simulink model "Project_SADC"  (R2021b)
settings: Solver=ode45  StartTime=0.0  StopTime=T  FixedStep=1e-6  RelTol=1e-12
values from neighbouring files (symbols this model uses):
  A = [A_sc,A_sp]    [Main_SADC_10572571.m]
  Abn0 = Anb0'    [Main_SADC_10572571.m]
  epsilon = deg2rad(23.45)    [Main_SADC_10572571.m]
  m = [0.01 0.05 0.01]'    [Main_SADC_10572571.m]
  N = [n1 n2 n3 n4 n5 n6 n7 n8 n9 n10]    [Main_SADC_10572571.m]
  n_sun = 2*pi / T_sun    (= 1.99238499086e-07)    [Main_SADC_10572571.m]
  P_srp = Fe_tot/c    [Main_SADC_10572571.m]
  R3H0 = data.Re^3*H0    [Main_SADC_10572571.m]
  R_sun = astroConstants(2)    [Main_SADC_10572571.m]
  rho_d = cat(2,ones(1,6)*rho_d_sc,ones(1,4)*rho_d_sp)    [Main_SADC_10572571.m]
  rho_s = cat(2,ones(1,6)*rho_s_sc,ones(1,4)*rho_s_sp)    [Main_SADC_10572571.m]
  ri = [ri_sc,r_sp1,r_sp1,r_sp2,r_sp2]    [Main_SADC_10572571.m]
  w0 = [wx0 wy0 wz0]'    [Main_SADC_10572571.m]
  weights = [0.15;0.5;0.35]    [Main_SADC_10572571.m]
undefined symbols (not defined in the file or in its folder): data, gyro, horizonsensor, magnetometer, rr0, sc, sunsensor, vv0, wheel
libraries: simulink_extras x10
(part 1 of 3)
settings Model: Creator=corra  LastModifiedBy=corra
settings SolverCC: AlgebraicLoopSolver=TrustRegion
settings DebuggingCC: SFMachineParentedDataDiag=warning

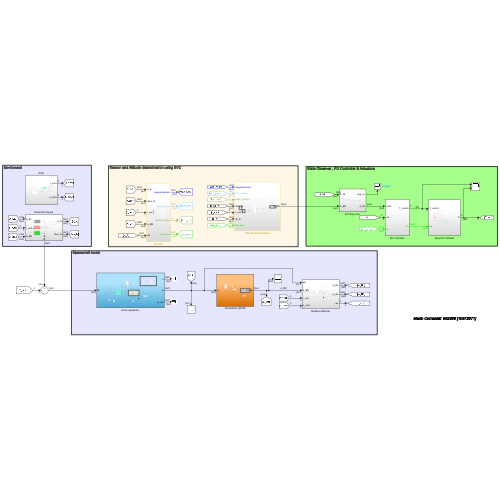
[thumbnail: Simulink's stored preview of the top-level diagram]
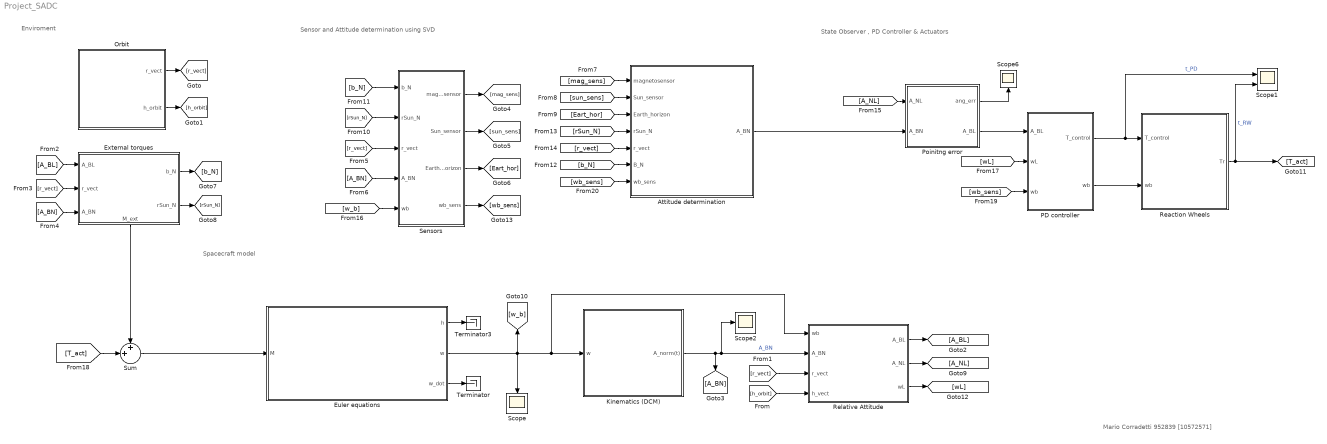
== system Project_SADC ==
  note: Mario Corradetti 952839 [10572571]
  note: Enviroment
  note: State Observer , PD Controller & Actuators
  note: Spacecraft model
  note: Sensor and Attitude determination using SVD
  "Attitude determination " : Subsystem
  Euler equations : Subsystem
  External torques : Subsystem
      settings: PortSchema="{\"entries\":[{\"content\":{\"sides\":[{\"content\":{\"connectorIds\":[\"In1\",\"In2\",\"In3\"]},\"type\":\"ConnectorPlacement.EquallySpacedRectSide\",\"uuid\":\"c5dd5657-11cd-46fc-a813-74747ea81146\"},{\"content\":{\"connectorIds\":[\"Out1\",\"Out2\"],\"side\":\"RIGHT\"},\"type\":\"ConnectorPlacement.EquallySpacedRectSide\",\"uuid\":\"ce8cbc86-0401-4f30-83b3-f262a6771dee\"},{\"content\":{\"connectorIds\":[],\"side\":\"TOP\"},\"type\":\"ConnectorPlacement.EquallySpacedRectSide\",\"uuid\":\"54f7f4d9-1155-478d-825b-4623d6763012\"},{\"content\":{\"connectorIds\":[\"Out3\"],\"side\":\"BOTTOM\"},\"type\":\"ConnectorPlacement.EquallySpacedRectSide\",\"uuid\":\"9bbeb954-f49a-41a5-9c63-5058200ec5df\"}]},\"type\":\"ConnectorPlacement.EquallySpacedConnector\",\"uuid\":\"ae160f86-5b24-4f86-a6f1-a9e1b48113ae\"}],\"packageUris\":[\"http://schema.mathworks.com/mf0/Connector/R2020b\"],\"version\":\"1.0\"}"
  Kinematics (DCM) : Subsystem
  Orbit : Subsystem
  PD controller : Subsystem
  Poinitng error : Subsystem
  Reaction Wheels : Subsystem
  Relative Attitude : Subsystem
  Scope : Scope
  Scope1 : Scope  NumInputPorts=2
  Scope2 : Scope
  Scope6 : Scope
  Sensors : Subsystem
  Sum : Sum  Inputs=++|
  Terminator : Terminator
  Terminator3 : Terminator
  wires:
  Euler equations/3(w_dot) -> Terminator/1
  Orbit/1(r_vect) -> [r_vect]
  Orbit/2(h_orbit) -> [h_orbit]
  Euler equations/1(h) -> Terminator3/1
  Kinematics (DCM)/1(A_norm(t)) -> Scope2/1, Relative Attitude/2(A_BN), [A_BN]  "A_BN"
  [r_vect] -> Relative Attitude/3(r_vect)
  [h_orbit] -> Relative Attitude/4(h_vect)
  Relative Attitude/1(A_BL) -> [A_BL]
  [A_BL] -> External torques/1(A_BL)
  [r_vect] -> External torques/2(r_vect)
  [A_BN] -> External torques/3(A_BN)
  [r_vect] -> Sensors/3(r_vect)
  [A_BN] -> Sensors/4(A_BN)
  Sensors/1(magnetosensor) -> [mag_sens]
  Sensors/2(Sun_sensor) -> [sun_sens]
  Sensors/3(Earth_horizon) -> [Eart_hor]
  [mag_sens] -> "Attitude determination "/1(magnetosensor)
  [sun_sens] -> "Attitude determination "/2(Sun_sensor)
  [Eart_hor] -> "Attitude determination "/3(Earth_horizon)
  External torques/1(b_N) -> [b_N]
  External torques/2(rSun_N) -> [rSun_N]
  [rSun_N] -> Sensors/2(rSun_N)
  [b_N] -> Sensors/1(b_N)
  [b_N] -> "Attitude determination "/6(" B_N ")
  [rSun_N] -> "Attitude determination "/4(rSun_N)
  [r_vect] -> "Attitude determination "/5(r_vect)
  Relative Attitude/2(A_NL) -> [A_NL]
  [A_NL] -> Poinitng error/1(A_NL)
  Poinitng error/1(ang_err) -> Scope6/1
  Poinitng error/2(A_BL) -> PD controller/1(A_BL)
  Euler equations/2(w) -> Scope/1, [w_b], Kinematics (DCM)/1(w), Relative Attitude/1(wb)
  [T_act] -> Sum/2
  Sum/1 -> Euler equations/1(M)
  External torques/3(M_ext) -> Sum/1
  PD controller/1(T_control) -> Reaction Wheels/1(T_control), Scope1/1  "t_PD"
  Relative Attitude/3(wL) -> [wL]
  [wL] -> PD controller/2(" wL ")
  PD controller/2(wb) -> Reaction Wheels/2(wb)
  [w_b] -> Sensors/5(wb)
  Sensors/4(wb_sens) -> [wb_sens]
  Reaction Wheels/1(Tr) -> [T_act], Scope1/2  "t_RW"
  [wb_sens] -> "Attitude determination "/7(wb_sens)
  "Attitude determination "/1(A_BN) -> Poinitng error/2(A_BN)
  [wb_sens] -> PD controller/3("wb ")

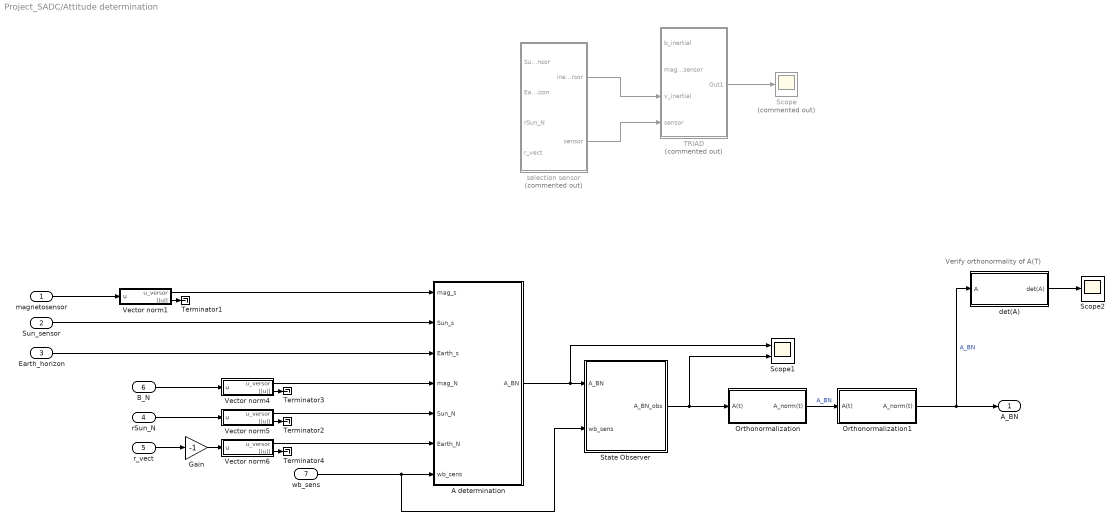
== system Project_SADC/Attitude determination  ==
  note: Verify orthonormality of A(T)
  magnetosensor : Inport
  Sun_sensor : Inport  Port=2
  Earth_horizon : Inport  Port=3
  rSun_N : Inport  Port=4
  r_vect : Inport  Port=5
  " B_N " : Inport  Port=6
  wb_sens : Inport  Port=7
  A determination : Subsystem
  Gain : Gain  Gain=-1
  Orthonormalization : Subsystem
  Orthonormalization1 : Subsystem
  Scope : Scope  Commented=on
  Scope1 : Scope  NumInputPorts=2
  Scope2 : Scope
  State Observer : Subsystem
  "TRIAD " : Subsystem  Commented=on
  Terminator{1..4} (4 alike) : Terminator
  Vector norm1 : Subsystem
  Vector norm4 : Subsystem
  Vector norm5 : Subsystem
  Vector norm6 : Subsystem
  det(A) : Subsystem
  selection sensor : Subsystem  Commented=on
  A_BN : Outport
  wires:
  r_vect/1 -> Gain/1
  magnetosensor/1 -> Vector norm1/1(u)
  Vector norm1/1(u_versor) -> A determination/1(mag_s)
  Sun_sensor/1 -> A determination/2(Sun_s)
  rSun_N/1 -> Vector norm5/1(u)
  Vector norm5/1(u_versor) -> A determination/5(Sun_N)
  Gain/1 -> Vector norm6/1(u)
  Vector norm6/1(u_versor) -> A determination/6(Earth_N)
  Vector norm1/2(||u||) -> Terminator1/1
  Vector norm4/2(||u||) -> Terminator3/1
  Vector norm5/2(||u||) -> Terminator2/1
  Vector norm6/2(||u||) -> Terminator4/1
  Orthonormalization/1(A_norm(t)) -> Orthonormalization1/1(A(t))  "A_BN"
  det(A)/1(det(A)) -> Scope2/1
  selection sensor/1(inertial versor) -> "TRIAD "/3(v_inertial)
  selection sensor/2(sensor) -> "TRIAD "/4(sensor)
  "TRIAD "/1(Out1) -> Scope/1
  " B_N "/1 -> Vector norm4/1(u)
  Vector norm4/1(u_versor) -> A determination/4(mag_N)
  Earth_horizon/1 -> A determination/3(Earth_s)
  wb_sens/1 -> State Observer/2(wb_sens), A determination/7(wb_sens)
  Orthonormalization1/1(A_norm(t)) -> A_BN/1, det(A)/1(A)  "A_BN"
  State Observer/1(A_BN_obs) -> Scope1/2, Orthonormalization/1(A(t))
  A determination/1(A_BN) -> Scope1/1, State Observer/1(A_BN)

== system Project_SADC/Euler equations ==
  note: INERTIA WHEEL
  note: Computation h vector of S/C
  M : Inport
  Clock1 : Clock
  Constant : Constant  Value=sc.I
  Constant1 : Constant  Value=sc.Iinv
  Constant2 : Constant  Value=wheel.I
  Constant3 : Constant  Value=wheel.w
  Gain : Gain  Gain=0
  Integrator : Integrator  InitialCondition=w0
  MatrixMultiply : Product  Multiplication=Matrix(*)
  Product : Product  Multiplication=Matrix(*)
  Product1 : Product  Multiplication=Matrix(*)
  Scope : Scope
  Scope1 : Scope
  Sum : Sum  Inputs=+-
  Sum1 : Sum
  Switch : Switch  Criteria=u2 > Threshold  Threshold=400
  To Workspace : ToWorkspace  VariableName=w  SaveFormat=Timeseries  SampleTime=-1
  product vector : Subsystem
  h : Outport
  w : Outport  Port=2
  w_dot : Outport  Port=3
  wires:
  Sum/1 -> Product1/2
  Product1/1 -> w_dot/1, Integrator/1  "w_dot"
  Product/1 -> h/1, Sum1/2  "h_B"
  Integrator/1 -> To Workspace/1, w/1, product vector/1(A), Product/2  "w"
  Constant1/1 -> Product1/1
  M/1 -> Sum/1  "external_moment & control_moment"
  Constant/1 -> Product/1
  product vector/1(C) -> Sum/2
  Constant2/1 -> MatrixMultiply/1
  Constant3/1 -> MatrixMultiply/2
  Sum1/1 -> Scope1/1, product vector/2(B)
  MatrixMultiply/1 -> Gain/1, Switch/1
  Gain/1 -> Switch/3
  Clock1/1 -> Switch/2
  Switch/1 -> Scope/1, Sum1/1

== system Project_SADC/External torques ==
  A_BL : Inport
  r_vect : Inport  Port=2
  A_BN : Inport  Port=3
  GG torque : Subsystem
  Gain : Gain
  Gain1 : Gain
  Gain2 : Gain
  Magnetic torque : Subsystem
  SRP torque : Subsystem
  Scope : Scope
  Scope1 : Scope
  Sum : Sum  Inputs=+++
  Terminator1 : Terminator
  Vector norm : Subsystem
  b_N : Outport
  rSun_N : Outport  Port=2
  M_ext : Outport  Port=3
  wires:
  A_BL/1 -> GG torque/1(A_BL)
  r_vect/1 -> Magnetic torque/2(r_vect), SRP torque/2(r_vect), GG torque/2(r_vect)
  A_BN/1 -> Magnetic torque/1(A_bn), SRP torque/1(A_BN)
  Sum/1 -> M_ext/1, Vector norm/1(u), Scope/1
  Magnetic torque/1(M_magnetic) -> Gain/1
  SRP torque/1(M_srp) -> Gain1/1
  GG torque/1(M_GG) -> Gain2/1
  Gain/1 -> Sum/1
  Gain1/1 -> Sum/2
  Gain2/1 -> Sum/3
  Magnetic torque/2(b_N) -> b_N/1
  SRP torque/2(rSun_N) -> rSun_N/1
  Vector norm/2(||u||) -> Scope1/1
  Vector norm/1(u_versor) -> Terminator1/1

== system Project_SADC/Kinematics (DCM) ==
  note: Verify orthonormality of A(T)
  w : Inport
  Gain : Gain  Gain=-1
  Integrator : Integrator  InitialCondition=Abn0
  Matrix Multiply : Product  Multiplication=Matrix(*)
  Orthonormalization : Subsystem
  Scope : Scope
  To Workspace : ToWorkspace  VariableName=A_bn  SaveFormat=Timeseries  SampleTime=-1
  det(A) : Subsystem
  w_mat : Subsystem
  A_norm(t) : Outport
  wires:
  w/1 -> w_mat/1(w)
  Matrix Multiply/1 -> Integrator/1  "A_dot"
  Gain/1 -> Matrix Multiply/1
  w_mat/1(w_mat) -> Gain/1
  Integrator/1 -> Orthonormalization/1(A(t))  "A(t)"
  Orthonormalization/1(A_norm(t)) -> det(A)/1(A), To Workspace/1, A_norm(t)/1, Matrix Multiply/2  "A_BN"
  det(A)/1(det(A)) -> Scope/1

== system Project_SADC/Orbit ==
  Constant : Constant  Value=[0 0 0]
  "Orbit integration " : Subsystem
  To Workspace : ToWorkspace  VariableName=h_orbit  SaveFormat=Timeseries  SampleTime=-1
  To Workspace2 : ToWorkspace  VariableName=r_orbit  SaveFormat=Timeseries  SampleTime=-1
  product vector : Subsystem
  r_vect : Outport
  h_orbit : Outport  Port=2
  wires:
  "Orbit integration "/1(r_vect) -> product vector/1(A), r_vect/1, To Workspace2/1
  "Orbit integration "/2(v_vect) -> product vector/2(B)
  Constant/1 -> "Orbit integration "/1(acc_pert)
  product vector/1(C) -> To Workspace/1, h_orbit/1

== system Project_SADC/PD controller ==
  A_BL : Inport
  " wL " : Inport  Port=2
  "wb " : Inport  Port=3
  Clock : Clock
  De-tumbling : Subsystem  TreatAsAtomicUnit=on
  If : If  IfExpression=u1<400
  If Action Subsystem : Subsystem  TreatAsAtomicUnit=on
  Merge : Merge
  T_control : Outport
  wb : Outport  Port=2
  wires:
  A_BL/1 -> If Action Subsystem/1(A_BL)
  If Action Subsystem/1(Output) -> Merge/1
  Merge/1 -> T_control/1
  "wb "/1 -> wb/1, De-tumbling/1(w_b), If Action Subsystem/3(w_b)
  If/1 -> De-tumbling/Action
  If/2 -> If Action Subsystem/Action
  De-tumbling/1(T_ideal) -> Merge/2
  Clock/1 -> If/1
  " wL "/1 -> If Action Subsystem/2("wL  ")

== system Project_SADC/Poinitng error ==
  A_NL : Inport
  A_BN : Inport  Port=2
  Acos : Trigonometry  Operator=acos
  Dot Product : DotProduct  InputSameDT=on  OutDataTypeStr=Inherit: Inherit via internal rule
  MatrixMultiply : Product  Multiplication=Matrix(*)
  MatrixMultiply1 : Product  Multiplication=Matrix(*)
  Radians to Degrees : simulink_extras/Transformations/Radians to Degrees
  To Workspace : ToWorkspace  VariableName=ang_err  SaveFormat=Timeseries  SampleTime=-1
  x_B : Constant  Value=[ 1 0 0 ]
  x_L : Constant  Value=[ 1 0 0 ]
  ang_err : Outport
  A_BL : Outport  Port=2
  wires:
  A_NL/1 -> MatrixMultiply/2
  A_BN/1 -> MatrixMultiply/1
  MatrixMultiply/1 -> A_BL/1, MatrixMultiply1/1  "A_BL"
  x_L/1 -> MatrixMultiply1/2
  MatrixMultiply1/1 -> Dot Product/1  "x_L in B"
  x_B/1 -> Dot Product/2
  Dot Product/1 -> Acos/1
  Acos/1 -> Radians to Degrees/1
  Radians to Degrees/1 -> To Workspace/1, ang_err/1

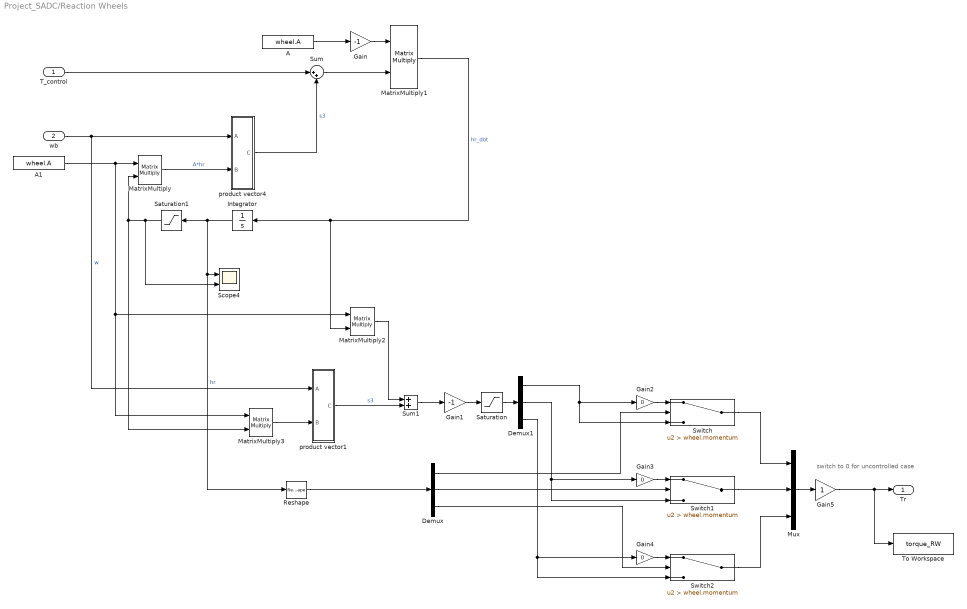
== system Project_SADC/Reaction Wheels ==
  note: switch to 0 for uncontrolled case
  T_control : Inport
  wb : Inport  Port=2
  A : Constant  Value=wheel.A
  A1 : Constant  Value=wheel.A
  Demux : Demux  Outputs=3
  Demux1 : Demux  Outputs=3
  Gain : Gain  Gain=-1
  Gain1 : Gain  Gain=-1
  Gain2 : Gain  Gain=0
  Gain3 : Gain  Gain=0
  Gain4 : Gain  Gain=0
  Gain5 : Gain
  Integrator : Integrator
  MatrixMultiply{,1..3} (4 alike) : Product  Multiplication=Matrix(*)
  Mux : Mux  Inputs=3
  Reshape : Reshape  OutputDimensionality=Column vector (2-D)
  Saturation : Saturate  UpperLimit=wheel.maxtorque  LowerLimit=-wheel.maxtorque  LinearizeAsGain=off
  Saturation1 : Saturate  UpperLimit=wheel.momentum  LowerLimit=-wheel.momentum
  Scope4 : Scope  NumInputPorts=2
  Sum : Sum  Inputs=|++
  Sum1 : Sum
  Switch : Switch  Criteria=u2 > Threshold  Threshold=wheel.momentum
  Switch1 : Switch  Criteria=u2 > Threshold  Threshold=wheel.momentum
  Switch2 : Switch  Criteria=u2 > Threshold  Threshold=wheel.momentum
  To Workspace : ToWorkspace  VariableName=torque_RW  SaveFormat=Timeseries  SampleTime=-1
  product vector1 : Subsystem
  product vector4 : Subsystem
  Tr : Outport
  wires:
  wb/1 -> product vector4/1(A), product vector1/1(A)  "w"
  MatrixMultiply/1 -> product vector4/2(B)  "A*hr"
  Integrator/1 -> Reshape/1, Scope4/1, Saturation1/1  "hr"
  T_control/1 -> Sum/1
  product vector4/1(C) -> Sum/2  "s3"
  MatrixMultiply1/1 -> Integrator/1, MatrixMultiply2/2  "hr_dot"
  Sum/1 -> MatrixMultiply1/2
  A1/1 -> MatrixMultiply3/1, MatrixMultiply2/1, MatrixMultiply/1
  A/1 -> Gain/1
  Gain/1 -> MatrixMultiply1/1
  MatrixMultiply2/1 -> Sum1/1
  product vector1/1(C) -> Sum1/2  "s3"
  Sum1/1 -> Gain1/1
  Gain1/1 -> Saturation/1
  Saturation1/1 -> Scope4/2, MatrixMultiply/2, MatrixMultiply3/2
  MatrixMultiply3/1 -> product vector1/2(B)
  Gain2/1 -> Switch/1
  Demux/1 -> Switch/2
  Gain3/1 -> Switch1/1
  Gain4/1 -> Switch2/1
  Demux/2 -> Switch1/2
  Demux/3 -> Switch2/2
  Switch/1 -> Mux/1
  Switch1/1 -> Mux/2
  Switch2/1 -> Mux/3
  Mux/1 -> Gain5/1
  Reshape/1 -> Demux/1
  Saturation/1 -> Demux1/1
  Demux1/1 -> Switch/3, Gain2/1
  Demux1/2 -> Switch1/3, Gain3/1
  Demux1/3 -> Switch2/3, Gain4/1
  Gain5/1 -> To Workspace/1, Tr/1

== system Project_SADC/Relative Attitude ==
  wb : Inport
  A_BN : Inport  Port=2
  r_vect : Inport  Port=3
  h_vect : Inport  Port=4
  DCM from L to B and from L to N : Subsystem
  MatrixMultiply : Product  Multiplication=Matrix(*)
  Scope : Scope
  Scope1 : Scope
  Sum : Sum  Inputs=-+
  A_BL : Outport
  A_NL : Outport  Port=2
  wL : Outport  Port=3
  wires:
  h_vect/1 -> DCM from L to B and from L to N/3(h_vect)
  DCM from L to B and from L to N/1(A_BL) -> A_BL/1, MatrixMultiply/1
  DCM from L to B and from L to N/2(A_NL) -> A_NL/1
  A_BN/1 -> DCM from L to B and from L to N/1(A_BN)
  Sum/1 -> Scope1/1  "w_B/L"
  r_vect/1 -> DCM from L to B and from L to N/2(r_vect)
  MatrixMultiply/1 -> Sum/1
  wb/1 -> Sum/2
  DCM from L to B and from L to N/3(wL) -> Scope/1, wL/1, MatrixMultiply/2

== system Project_SADC/Sensors ==
  b_N : Inport
  rSun_N : Inport  Port=2
  r_vect : Inport  Port=3
  A_BN : Inport  Port=4
  wb : Inport  Port=5
  Check if in EH FOV : Subsystem
  Check if in sunsensor FOV : Subsystem
  Cylindrical eclipse model : Subsystem  Commented=on
  Earth horizon : Subsystem
  Gyroscope : Subsystem
  Magnetosensor : Subsystem
  MatrixMultiply1 : Product  Multiplication=Matrix(*)
  Scope4 : Scope  NumInputPorts=2
  Scope5 : Scope  NumInputPorts=2
  Scope6 : Scope  NumInputPorts=2
  Sun sensor : Subsystem
  magnetosensor : Outport
  Sun_sensor : Outport  Port=2
  Earth_horizon : Outport  Port=3
  wb_sens : Outport  Port=4
  wires:
  A_BN/1 -> Check if in EH FOV/1(A_BN), MatrixMultiply1/1, Check if in sunsensor FOV/2(A_BN)
  r_vect/1 -> Check if in sunsensor FOV/3(r_vect), Check if in EH FOV/2(r_vect)
  Magnetosensor/1(b_measured) -> Scope4/2, magnetosensor/1
  rSun_N/1 -> Check if in sunsensor FOV/1(rSun_N)
  b_N/1 -> MatrixMultiply1/2
  MatrixMultiply1/1 -> Scope4/1, Magnetosensor/1(b_B)
  Check if in sunsensor FOV/2(rSun_B) -> Sun sensor/1(rSun_B)  "r_sun_B"
  Sun sensor/1(Output1) -> Scope5/2, Sun_sensor/1
  Earth horizon/1(Output2) -> Earth_horizon/1, Scope6/2  "sens"
  wb/1 -> Gyroscope/1(wb)
  Gyroscope/1(w_sens) -> wb_sens/1
  Check if in sunsensor FOV/1(Sun_B) -> Scope5/1
  Check if in EH FOV/1(rvect _B) -> Scope6/1, Earth horizon/1(rEarth_B)  "r_Earth_B"

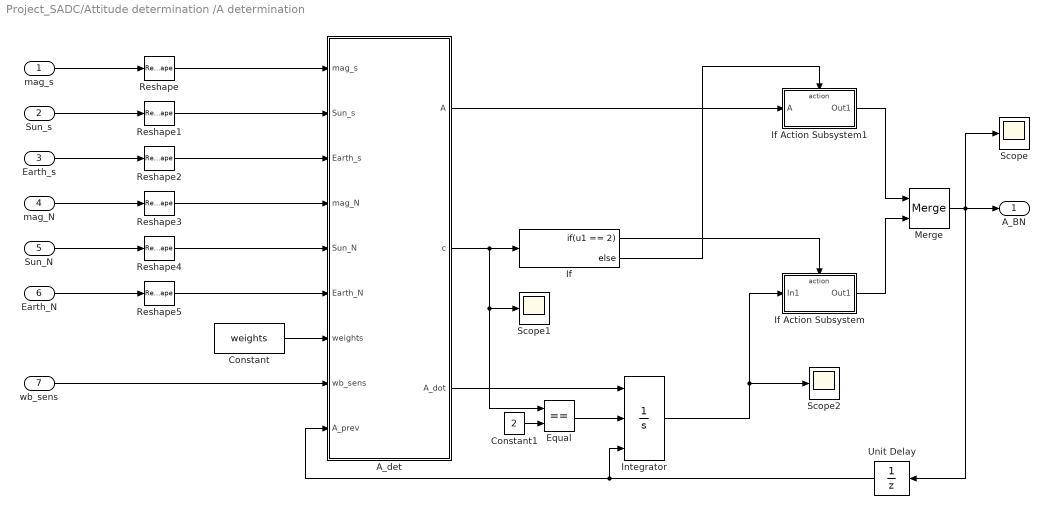
== system Project_SADC/Attitude determination /A determination ==
  mag_s : Inport
  Sun_s : Inport  Port=2
  Earth_s : Inport  Port=3
  mag_N : Inport  Port=4
  Sun_N : Inport  Port=5
  Earth_N : Inport  Port=6
  wb_sens : Inport  Port=7
  A_det : MATLAB Function  TreatAsAtomicUnit=on
  Constant : Constant  Value=weights  VectorParams1D=off
  Constant1 : Constant  Value=2
  Equal : RelationalOperator  Operator===  OutDataTypeStr=boolean  RndMeth=Simplest
  If : If  IfExpression=u1 == 2
  If Action Subsystem : Subsystem  TreatAsAtomicUnit=on
  If Action Subsystem1 : Subsystem  TreatAsAtomicUnit=on
  Integrator : Integrator  ExternalReset=either  InitialConditionSource=external  InitialCondition=eye(3)
  Merge : Merge
  Reshape{,1..5} (6 alike) : Reshape  OutputDimensionality=Column vector (2-D)
  Scope : Scope
  Scope1 : Scope
  Scope2 : Scope
  Unit Delay : UnitDelay  InitialCondition=Abn0  SampleTime=-1  HasFrameUpgradeWarning=on
  A_BN : Outport
  wires:
  mag_s/1 -> Reshape/1
  Sun_s/1 -> Reshape1/1
  Earth_s/1 -> Reshape2/1
  mag_N/1 -> Reshape3/1
  Sun_N/1 -> Reshape4/1
  Earth_N/1 -> Reshape5/1
  Constant/1 -> A_det/7(weights)
  Reshape/1 -> A_det/1(mag_s)
  Reshape1/1 -> A_det/2(Sun_s)
  Reshape2/1 -> A_det/3(Earth_s)
  Reshape3/1 -> A_det/4(mag_N)
  Reshape4/1 -> A_det/5(Sun_N)
  Reshape5/1 -> A_det/6(Earth_N)
  wb_sens/1 -> A_det/8(wb_sens)
  A_det/3(A_dot) -> Integrator/1
  Integrator/1 -> Scope2/1, If Action Subsystem/1(In1)
  A_det/2(c) -> Scope1/1, Equal/1, If/1
  If/1 -> If Action Subsystem/Action
  If/2 -> If Action Subsystem1/Action
  Merge/1 -> Unit Delay/1, Scope/1, A_BN/1
  Equal/1 -> Integrator/2
  Constant1/1 -> Equal/2
  Unit Delay/1 -> A_det/9(A_prev), Integrator/3
  A_det/1(A) -> If Action Subsystem1/1(A)
  If Action Subsystem/1(Out1) -> Merge/2
  If Action Subsystem1/1(Out1) -> Merge/1

== system Project_SADC/Attitude determination /Orthonormalization ==
  A(t) : Inport
  Gain : Gain  Gain=3/2
  Gain1 : Gain  Gain=1/2
  Matrix Multiply : Product  Multiplication=Matrix(*)
  Matrix Multiply1 : Product  Multiplication=Matrix(*)
  Sum : Sum  Inputs=+-
  Transpose : Math  Operator=transpose  SaturateOnIntegerOverflow=on
  A_norm(t) : Outport
  wires:
  Gain/1 -> Sum/1
  Transpose/1 -> Matrix Multiply/2
  A(t)/1 -> Gain/1, Gain1/1, Transpose/1, Matrix Multiply/1
  Matrix Multiply1/1 -> Sum/2
  Sum/1 -> A_norm(t)/1
  Matrix Multiply/1 -> Matrix Multiply1/1
  Gain1/1 -> Matrix Multiply1/2

== system Project_SADC/Attitude determination /Orthonormalization1 ==
  A(t) : Inport
  Gain : Gain  Gain=3/2
  Gain1 : Gain  Gain=1/2
  Matrix Multiply : Product  Multiplication=Matrix(*)
  Matrix Multiply1 : Product  Multiplication=Matrix(*)
  Sum : Sum  Inputs=+-
  Transpose : Math  Operator=transpose  SaturateOnIntegerOverflow=on
  A_norm(t) : Outport
  wires:
  Gain1/1 -> Matrix Multiply1/2
  Matrix Multiply/1 -> Matrix Multiply1/1
  Sum/1 -> A_norm(t)/1
  Matrix Multiply1/1 -> Sum/2
  A(t)/1 -> Matrix Multiply/1, Transpose/1, Gain1/1, Gain/1
  Transpose/1 -> Matrix Multiply/2
  Gain/1 -> Sum/1

== system Project_SADC/Attitude determination /State Observer ==
  A_BN : Inport
  wb_sens : Inport  Port=2
  Gain : Gain  Gain=-0.6
  Gain1 : Gain  Gain=+1
  Integrator1 : Integrator  InitialCondition=Abn0
  MatrixMultiply : Product  Multiplication=Matrix(*)
  Scope : Scope  NumInputPorts=2
  Subsystem : Subsystem
  Sum : Sum  Inputs=|++
  Sum1 : Sum  Inputs=+-
  A_BN_obs : Outport
  wires:
  Integrator1/1 -> Scope/1, A_BN_obs/1, MatrixMultiply/2, Sum1/1  "ABN_obs"
  Subsystem/1(skew_mat) -> Gain1/1
  A_BN/1 -> Scope/2, Sum1/2  "ABN_sens"
  Sum1/1 -> Gain/1
  MatrixMultiply/1 -> Sum/1
  Gain/1 -> Sum/2
  Sum/1 -> Integrator1/1
  wb_sens/1 -> Subsystem/1(vect)  "wb_obs"
  Gain1/1 -> MatrixMultiply/1

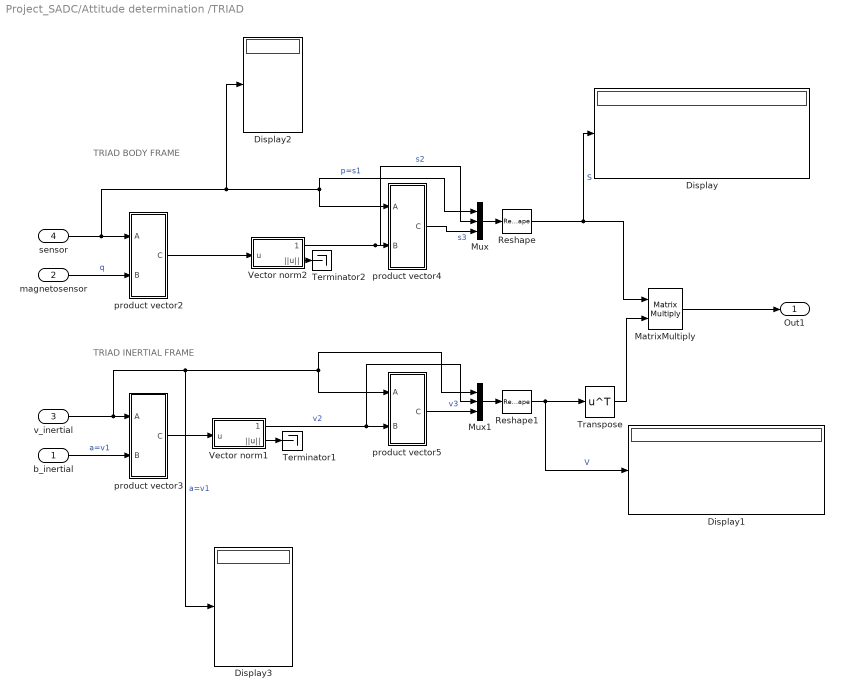
== system Project_SADC/Attitude determination /TRIAD  ==
  note: TRIAD BODY FRAME
  note: TRIAD INERTIAL FRAME
  b_inertial : Inport
  magnetosensor : Inport  Port=2
  v_inertial : Inport  Port=3
  sensor : Inport  Port=4
  Display{,1..3} (4 alike) : Display
  MatrixMultiply : Product  Multiplication=Matrix(*)
  Mux : Mux  Inputs=3
  Mux1 : Mux  Inputs=3
  Reshape : Reshape  OutputDimensionality=Customize  OutputDimensions=[3,3]
  Reshape1 : Reshape  OutputDimensionality=Customize  OutputDimensions=[3,3]
  Terminator1 : Terminator
  Terminator2 : Terminator
  Transpose : Math  Operator=transpose  SaturateOnIntegerOverflow=on
  Vector norm1 : Subsystem
  Vector norm2 : Subsystem
  product vector2 : Subsystem
  product vector3 : Subsystem
  product vector4 : Subsystem
  product vector5 : Subsystem
  Out1 : Outport
  wires:
  sensor/1 -> Display2/1, Mux/1, product vector4/1(A), product vector2/1(A)  "p=s1"
  magnetosensor/1 -> product vector2/2(B)  "q"
  v_inertial/1 -> Display3/1, Mux1/1, product vector5/1(A), product vector3/1(A)  "a=v1"
  product vector2/1(C) -> Vector norm2/1(u)
  product vector3/1(C) -> Vector norm1/1(u)
  Vector norm2/1(u_versor) -> Mux/2, product vector4/2(B)  "s2"
  Vector norm1/1(u_versor) -> Mux1/2, product vector5/2(B)  "v2"
  product vector5/1(C) -> Mux1/3  "v3"
  product vector4/1(C) -> Mux/3  "s3"
  Mux/1 -> Reshape/1
  Mux1/1 -> Reshape1/1
  Reshape/1 -> Display/1, MatrixMultiply/1  "S"
  Reshape1/1 -> Display1/1, Transpose/1  "V"
  MatrixMultiply/1 -> Out1/1
  Transpose/1 -> MatrixMultiply/2
  Vector norm2/2(||u||) -> Terminator2/1
  Vector norm1/2(||u||) -> Terminator1/1
  b_inertial/1 -> product vector3/2(B)  "a=v1"

== system Project_SADC/Attitude determination /Vector norm1 ==
  u : Inport
  Divide : Product  Inputs=*/
  norm_vector : Subsystem
  u_versor : Outport
  ||u|| : Outport  Port=2
  wires:
  u/1 -> Divide/1, norm_vector/1(u)
  norm_vector/1(|u|) -> ||u||/1, Divide/2
  Divide/1 -> u_versor/1

== system Project_SADC/Attitude determination /Vector norm4 ==
  u : Inport
  Divide : Product  Inputs=*/
  norm_vector : Subsystem
  u_versor : Outport
  ||u|| : Outport  Port=2
  wires:
  u/1 -> Divide/1, norm_vector/1(u)
  norm_vector/1(|u|) -> ||u||/1, Divide/2
  Divide/1 -> u_versor/1

== system Project_SADC/Attitude determination /Vector norm5 ==
  u : Inport
  Divide : Product  Inputs=*/
  norm_vector : Subsystem
  u_versor : Outport
  ||u|| : Outport  Port=2
  wires:
  Divide/1 -> u_versor/1
  norm_vector/1(|u|) -> Divide/2, ||u||/1
  u/1 -> norm_vector/1(u), Divide/1

== system Project_SADC/Attitude determination /Vector norm6 ==
  u : Inport
  Divide : Product  Inputs=*/
  norm_vector : Subsystem
  u_versor : Outport
  ||u|| : Outport  Port=2
  wires:
  u/1 -> Divide/1, norm_vector/1(u)
  norm_vector/1(|u|) -> ||u||/1, Divide/2
  Divide/1 -> u_versor/1

== system Project_SADC/Attitude determination /det(A) ==
  A : Inport
  Demux : Demux  Outputs=9
  Product{,1..8} (9 alike) : Product
  Reshape : Reshape  OutputDimensionality=Customize  OutputDimensions=[9,1]
  Sum : Sum  Inputs=+-
  Sum1 : Sum  Inputs=+-+
  Sum2 : Sum  Inputs=+-
  Sum3 : Sum  Inputs=+-
  det(A) : Outport
  wires:
  Product/1 -> Sum/1
  Demux/5 -> Product7/1, Product/1  "a22"
  Demux/9 -> Product3/2, Product/2  "a33"
  Demux/6 -> Product1/1, Product4/2  "a23"
  Demux/8 -> Product1/2, Product6/2  "a32"
  Product1/1 -> Sum/2
  Demux/1 -> Product2/2  "a11"
  Sum/1 -> Product2/1
  Demux/4 -> Product6/1, Product3/1  "a21"
  Demux/7 -> Product7/2, Product4/1  "a31"
  Product3/1 -> Sum2/1
  Product4/1 -> Sum2/2
  Sum2/1 -> Product5/2
  Demux/2 -> Product5/1  "a12"
  Product2/1 -> Sum1/1
  Product5/1 -> Sum1/2
  Product6/1 -> Sum3/1
  Product7/1 -> Sum3/2
  Sum3/1 -> Product8/2
  Demux/3 -> Product8/1  "a13"
  Product8/1 -> Sum1/3
  Sum1/1 -> det(A)/1
  Reshape/1 -> Demux/1
  A/1 -> Reshape/1

== system Project_SADC/Attitude determination /selection sensor ==
  Sun_sensor : Inport
  Earth_horizon : Inport  Port=2
  rSun_N : Inport  Port=3
  r_vect : Inport  Port=4
  If : If  IfExpression=u1==0
  If Action Subsystem : Subsystem  TreatAsAtomicUnit=on
  If Action Subsystem1 : Subsystem  TreatAsAtomicUnit=on
  If Action Subsystem2 : Subsystem  TreatAsAtomicUnit=on
  If Action Subsystem3 : Subsystem  TreatAsAtomicUnit=on
  If1 : If  IfExpression=u1==0
  Merge : Merge
  Merge1 : Merge
  Terminator : Terminator
  Vector norm3 : Subsystem
  inertial versor : Outport
  sensor : Outport  Port=2
  wires:
  Sun_sensor/1 -> If Action Subsystem1/1(Sun_sensor), Vector norm3/1(u)
  If/1 -> If Action Subsystem/Action
  If/2 -> If Action Subsystem1/Action
  Earth_horizon/1 -> If Action Subsystem/1(Earth_horizon)
  Vector norm3/2(||u||) -> If1/1, If/1
  Vector norm3/1(u_versor) -> Terminator/1
  If Action Subsystem1/1(Out1) -> Merge/2
  If Action Subsystem/1(Out1) -> Merge/1
  Merge/1 -> sensor/1
  r_vect/1 -> If Action Subsystem2/1(r_vect)
  rSun_N/1 -> If Action Subsystem3/1(In1)
  If Action Subsystem2/1(Out1) -> Merge1/1
  If Action Subsystem3/1(Out1) -> Merge1/2
  Merge1/1 -> inertial versor/1
  If1/1 -> If Action Subsystem2/Action
  If1/2 -> If Action Subsystem3/Action

== system Project_SADC/Euler equations/product vector ==
  A : Inport
  B : Inport  Port=2
  Mux : Mux  Inputs=3
  i-component : Subsystem
  j-component : Subsystem
  k-component1 : Subsystem
  C : Outport
  wires:
  Mux/1 -> C/1
  A/1 -> k-component1/1(A), j-component/1(A), i-component/1(A)
  B/1 -> k-component1/2(B), j-component/2(B), i-component/2(B)
  i-component/1(Out2) -> Mux/1
  j-component/1(Out1) -> Mux/2
  k-component1/1(Out1) -> Mux/3

== system Project_SADC/External torques/GG torque ==
  A_BL : Inport
  r_vect : Inport  Port=2
  Constant : Constant  Value=-3
  Constant1 : Constant  Value=[1 0 0]'  VectorParams1D=off
  Constant2 : Constant  Value=sc.I  VectorParams1D=off
  Gain : Gain  Gain=data.mu*3
  MatrixMultiply : Product  Multiplication=Matrix(*)
  MatrixMultiply1 : Product  Multiplication=Matrix(*)
  MatrixMultiply2 : Product  Multiplication=Matrix(*)
  Power : Math  Operator=pow  SaturateOnIntegerOverflow=on
  Reshape : Reshape  OutputDimensionality=Column vector (2-D)
  Scope : Scope
  Terminator : Terminator
  To Workspace : ToWorkspace  VariableName=M_GG  SaveFormat=Timeseries  SampleTime=-1
  Vector norm : Subsystem
  product vector : Subsystem
  M_GG : Outport
  wires:
  r_vect/1 -> Vector norm/1(u)
  Vector norm/1(u_versor) -> Terminator/1
  Vector norm/2(||u||) -> Power/1
  Constant/1 -> Power/2
  Power/1 -> Gain/1
  A_BL/1 -> MatrixMultiply/1
  Constant1/1 -> MatrixMultiply/2
  MatrixMultiply/1 -> product vector/1(A), MatrixMultiply1/2  "[c1,c2,c3]'"
  Constant2/1 -> MatrixMultiply1/1
  MatrixMultiply1/1 -> product vector/2(B)
  Gain/1 -> MatrixMultiply2/2
  product vector/1(C) -> MatrixMultiply2/1
  MatrixMultiply2/1 -> Reshape/1
  Reshape/1 -> To Workspace/1, Scope/1, M_GG/1

== system Project_SADC/External torques/Magnetic torque ==
  A_bn : Inport
  r_vect : Inport  Port=2
  Clock : Clock
  Constant : Constant  Value=m
  MatrixMultiply : Product  Multiplication=Matrix(*)
  Reshape : Reshape  OutputDimensionality=Column vector (2-D)
  Scope : Scope
  To Workspace : ToWorkspace  VariableName=M_magnetic  SaveFormat=Timeseries  SampleTime=-1
  mag_field in inertial : Subsystem
  product vector2 : Subsystem
  M_magnetic : Outport
  b_N : Outport  Port=2
  wires:
  r_vect/1 -> mag_field in inertial/1(r_vect)
  Clock/1 -> mag_field in inertial/2(time)
  mag_field in inertial/1(b_B) -> b_N/1, MatrixMultiply/2
  A_bn/1 -> MatrixMultiply/1
  MatrixMultiply/1 -> product vector2/2(B)  "magnetic vector in body frame"
  Constant/1 -> product vector2/1(A)
  product vector2/1(C) -> Reshape/1
  Reshape/1 -> To Workspace/1, Scope/1, M_magnetic/1

== system Project_SADC/External torques/SRP torque ==
  A_BN : Inport
  r_vect : Inport  Port=2
  Clock : Clock
  Display : Display
  SRP forces : Subsystem
  Scope : Scope
  Scope1 : Scope
  Sun wrt s/c : Subsystem
  To Workspace : ToWorkspace  VariableName=M_srp  SaveFormat=Timeseries  SampleTime=-1
  Torques on faces of s/c : Subsystem
  M_srp : Outport
  rSun_N : Outport  Port=2
  wires:
  A_BN/1 -> Sun wrt s/c/1(A_BN)
  r_vect/1 -> Sun wrt s/c/2(r_vect)
  Clock/1 -> Sun wrt s/c/3(t)
  Sun wrt s/c/1(r_sun) -> Display/1, SRP forces/1(r_Sun)  "r_Sun_in_body"
  SRP forces/2(S_dot_N) -> Torques on faces of s/c/2(S_N)
  SRP forces/1(F_srp) -> Torques on faces of s/c/1(F_srp), Scope/1
  Sun wrt s/c/2(rSun_N) -> rSun_N/1
  Torques on faces of s/c/1(M_srp) -> Scope1/1, To Workspace/1, M_srp/1  "M_srp"

== system Project_SADC/External torques/Vector norm ==
  u : Inport
  Divide : Product  Inputs=*/
  norm_vector : Subsystem
  u_versor : Outport
  ||u|| : Outport  Port=2
  wires:
  u/1 -> Divide/1, norm_vector/1(u)
  norm_vector/1(|u|) -> ||u||/1, Divide/2
  Divide/1 -> u_versor/1

== system Project_SADC/Kinematics (DCM)/Orthonormalization ==
  A(t) : Inport
  Gain : Gain  Gain=3/2
  Gain1 : Gain  Gain=1/2
  Matrix Multiply : Product  Multiplication=Matrix(*)
  Matrix Multiply1 : Product  Multiplication=Matrix(*)
  Sum : Sum  Inputs=+-
  Transpose : Math  Operator=transpose  SaturateOnIntegerOverflow=on
  A_norm(t) : Outport
  wires:
  Gain/1 -> Sum/1
  Transpose/1 -> Matrix Multiply/2
  A(t)/1 -> Gain/1, Gain1/1, Transpose/1, Matrix Multiply/1
  Matrix Multiply1/1 -> Sum/2
  Sum/1 -> A_norm(t)/1
  Matrix Multiply/1 -> Matrix Multiply1/1
  Gain1/1 -> Matrix Multiply1/2

== system Project_SADC/Kinematics (DCM)/det(A) ==
  A : Inport
  Demux : Demux  Outputs=9
  Product{,1..8} (9 alike) : Product
  Reshape : Reshape  OutputDimensionality=Customize  OutputDimensions=[9,1]
  Sum : Sum  Inputs=+-
  Sum1 : Sum  Inputs=+-+
  Sum2 : Sum  Inputs=+-
  Sum3 : Sum  Inputs=+-
  det(A) : Outport
  wires:
  Product/1 -> Sum/1
  Demux/5 -> Product7/1, Product/1  "a22"
  Demux/9 -> Product3/2, Product/2  "a33"
  Demux/6 -> Product1/1, Product4/2  "a23"
  Demux/8 -> Product1/2, Product6/2  "a32"
  Product1/1 -> Sum/2
  Demux/1 -> Product2/2  "a11"
  Sum/1 -> Product2/1
  Demux/4 -> Product6/1, Product3/1  "a21"
  Demux/7 -> Product7/2, Product4/1  "a31"
  Product3/1 -> Sum2/1
  Product4/1 -> Sum2/2
  Sum2/1 -> Product5/2
  Demux/2 -> Product5/1  "a12"
  Product2/1 -> Sum1/1
  Product5/1 -> Sum1/2
  Product6/1 -> Sum3/1
  Product7/1 -> Sum3/2
  Sum3/1 -> Product8/2
  Demux/3 -> Product8/1  "a13"
  Product8/1 -> Sum1/3
  Sum1/1 -> det(A)/1
  Reshape/1 -> Demux/1
  A/1 -> Reshape/1

== system Project_SADC/Kinematics (DCM)/w_mat ==
  w : Inport
  Constant : Constant  Value=0
  Constant1 : Constant  Value=0
  Constant7 : Constant  Value=0
  Demux : Demux  Outputs=3
  Gain1 : Gain  Gain=-1
  Gain2 : Gain  Gain=-1
  Gain3 : Gain  Gain=-1
  Mux : Mux  Inputs=9
  Reshape : Reshape  OutputDimensionality=Customize  OutputDimensions=[3,3]
  Transpose : Math  Operator=transpose  SaturateOnIntegerOverflow=on
  w_mat : Outport
  wires:
  Gain3/1 -> Mux/7
  Demux/2 -> Mux/3, Gain3/1
  Demux/3 -> Mux/4, Gain2/1
  Constant7/1 -> Mux/9
  Demux/1 -> Mux/8, Gain1/1
  Constant/1 -> Mux/1
  Mux/1 -> Reshape/1
  Constant1/1 -> Mux/5
  Gain2/1 -> Mux/2
  Gain1/1 -> Mux/6
  w/1 -> Demux/1
  Reshape/1 -> Transpose/1
  Transpose/1 -> w_mat/1

== system Project_SADC/Orbit/Orbit integration  ==
  acc_pert : Inport
  Constant : Constant  Value=-3
  Gain : Gain  Gain=- data.mu
  Integrator : Integrator  InitialCondition=vv0
  Integrator1 : Integrator  InitialCondition=rr0
  MatrixMultiply : Product
  Power : Math  Operator=pow  SaturateOnIntegerOverflow=on
  Subsystem1 : Subsystem
  Sum : Sum  Inputs=|++
  Terminator : Terminator
  r_vect : Outport
  v_vect : Outport  Port=2
  wires:
  Integrator/1 -> v_vect/1, Integrator1/1  "v"
  Integrator1/1 -> MatrixMultiply/1, Subsystem1/1(u), r_vect/1  "r"
  acc_pert/1 -> Sum/1
  Sum/1 -> Integrator/1  "a"
  Gain/1 -> Sum/2
  Subsystem1/2(||u||) -> Power/1  "||r||"
  Subsystem1/1(u_versor) -> Terminator/1
  Constant/1 -> Power/2
  MatrixMultiply/1 -> Gain/1
  Power/1 -> MatrixMultiply/2  "||r||^-3"

== system Project_SADC/Orbit/product vector ==
  A : Inport
  B : Inport  Port=2
  Mux : Mux  Inputs=3
  i-component : Subsystem
  j-component : Subsystem
  k-component1 : Subsystem
  C : Outport
  wires:
  Mux/1 -> C/1
  A/1 -> k-component1/1(A), j-component/1(A), i-component/1(A)
  B/1 -> k-component1/2(B), j-component/2(B), i-component/2(B)
  i-component/1(Out2) -> Mux/1
  j-component/1(Out1) -> Mux/2
  k-component1/1(Out1) -> Mux/3

== system Project_SADC/PD controller/De-tumbling ==
  note: Proportional
  w_b : Inport
  Action Port : ActionPort  ActionPortLabel=if(u1<400)
  Demux : Demux  Outputs=3
  Mux2 : Mux  Inputs=3
  kd1 : Gain  Gain=-1e-3
  kd2 : Gain  Gain=-1e-3
  kp : Gain  Gain=-1e-3
  T_ideal : Outport
  wires:
  Demux/1 -> kd2/1
  kd2/1 -> Mux2/1
  kp/1 -> Mux2/3
  Demux/2 -> kd1/1
  Demux/3 -> kp/1
  kd1/1 -> Mux2/2
  w_b/1 -> Demux/1
  Mux2/1 -> T_ideal/1

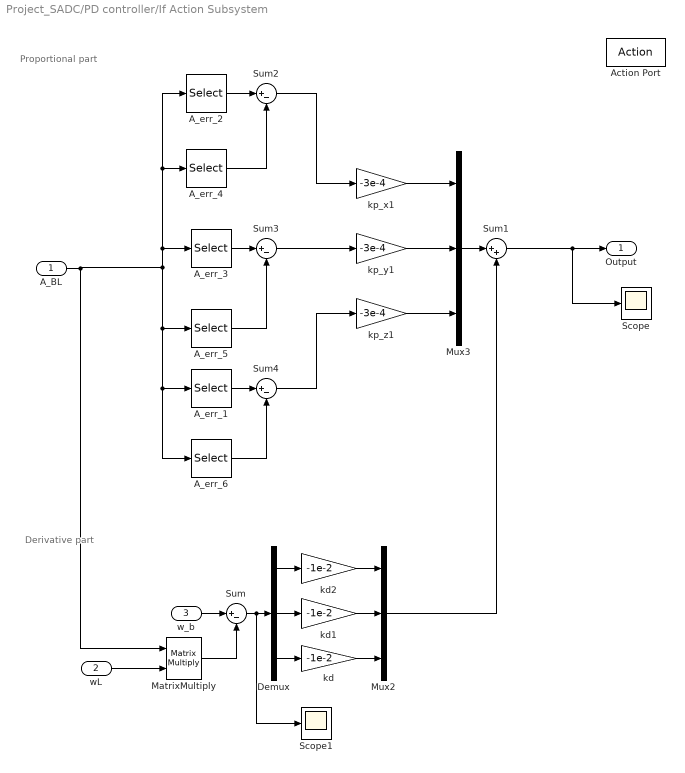
== system Project_SADC/PD controller/If Action Subsystem ==
  note: Derivative part
  note: Proportional part
  A_BL : Inport
  "wL  " : Inport  Port=2
  w_b : Inport  Port=3
  Action Port : ActionPort  ActionPortLabel=else
  A_err_1 : Selector  NumberOfDimensions=2  InputPortWidth=3  IndexOptions=Index vector (dialog),Index vector (dialog)  Indices=1,2  OutputSizes=1,1
  A_err_2 : Selector  NumberOfDimensions=2  InputPortWidth=3  IndexOptions=Index vector (dialog),Index vector (dialog)  Indices=2,3  OutputSizes=1,1
  A_err_3 : Selector  NumberOfDimensions=2  InputPortWidth=3  IndexOptions=Index vector (dialog),Index vector (dialog)  Indices=3,1  OutputSizes=1,1
  A_err_4 : Selector  NumberOfDimensions=2  InputPortWidth=3  IndexOptions=Index vector (dialog),Index vector (dialog)  Indices=3,2  OutputSizes=1,1
  A_err_5 : Selector  NumberOfDimensions=2  InputPortWidth=3  IndexOptions=Index vector (dialog),Index vector (dialog)  Indices=1,3  OutputSizes=1,1
  A_err_6 : Selector  NumberOfDimensions=2  InputPortWidth=3  IndexOptions=Index vector (dialog),Index vector (dialog)  Indices=2,1  OutputSizes=1,1
  Demux : Demux  Outputs=3
  MatrixMultiply : Product  Multiplication=Matrix(*)
  Mux2 : Mux  Inputs=3
  Mux3 : Mux  Inputs=3
  Scope : Scope
  Scope1 : Scope
  Sum{,2..4} (4 alike) : Sum  Inputs=|+-
  Sum1 : Sum  Inputs=|++
  kd : Gain  Gain=-1e-2
  kd1 : Gain  Gain=-1e-2
  kd2 : Gain  Gain=-1e-2
  kp_x1 : Gain  Gain=-3e-4
  kp_y1 : Gain  Gain=-3e-4
  kp_z1 : Gain  Gain=-3e-4
  Output : Outport
  wires:
  MatrixMultiply/1 -> Sum/2
  kd/1 -> Mux2/3
  kd1/1 -> Mux2/2
  Demux/1 -> kd2/1
  Mux2/1 -> Sum1/2
  Demux/3 -> kd/1
  w_b/1 -> Sum/1
  Sum/1 -> Scope1/1, Demux/1
  kd2/1 -> Mux2/1
  Demux/2 -> kd1/1
  "wL  "/1 -> MatrixMultiply/2
  Sum1/1 -> Output/1, Scope/1
  kp_x1/1 -> Mux3/1
  kp_y1/1 -> Mux3/2
  kp_z1/1 -> Mux3/3
  A_BL/1 -> A_err_4/1, A_err_2/1, A_err_3/1, A_err_5/1, A_err_6/1, A_err_1/1, MatrixMultiply/1
  Mux3/1 -> Sum1/1
  A_err_2/1 -> Sum2/1
  A_err_4/1 -> Sum2/2
  A_err_3/1 -> Sum3/1
  A_err_5/1 -> Sum3/2
  A_err_1/1 -> Sum4/1
  A_err_6/1 -> Sum4/2
  Sum2/1 -> kp_x1/1
  Sum3/1 -> kp_y1/1
  Sum4/1 -> kp_z1/1

== system Project_SADC/Reaction Wheels/product vector1 ==
  A : Inport
  B : Inport  Port=2
  Mux : Mux  Inputs=3
  i-component : Subsystem
  j-component : Subsystem
  k-component1 : Subsystem
  C : Outport
  wires:
  k-component1/1(Out1) -> Mux/3
  j-component/1(Out1) -> Mux/2
  i-component/1(Out2) -> Mux/1
  B/1 -> i-component/2(B), j-component/2(B), k-component1/2(B)
  A/1 -> i-component/1(A), j-component/1(A), k-component1/1(A)
  Mux/1 -> C/1

== system Project_SADC/Reaction Wheels/product vector4 ==
  A : Inport
  B : Inport  Port=2
  Mux : Mux  Inputs=3
  i-component : Subsystem
  j-component : Subsystem
  k-component1 : Subsystem
  C : Outport
  wires:
  Mux/1 -> C/1
  A/1 -> k-component1/1(A), j-component/1(A), i-component/1(A)
  B/1 -> k-component1/2(B), j-component/2(B), i-component/2(B)
  i-component/1(Out2) -> Mux/1
  j-component/1(Out1) -> Mux/2
  k-component1/1(Out1) -> Mux/3

== system Project_SADC/Relative Attitude/DCM from L to B and from L to N ==
  A_BN : Inport
  r_vect : Inport  Port=2
  h_vect : Inport  Port=3
  DCM from L to N : Subsystem
  Divide : Product  Inputs=*/
  Gain : Gain  Gain=[ 0 0 1]
  MatrixMultiply : Product  Multiplication=Matrix(*)
  Square : Math  Operator=square  SaturateOnIntegerOverflow=on
  Terminator1 : Terminator
  Terminator2 : Terminator
  To Workspace : ToWorkspace  VariableName=A_nl  SaveFormat=Timeseries  SampleTime=-1
  Vector norm : Subsystem
  Vector norm1 : Subsystem
  A_BL : Outport
  A_NL : Outport  Port=2
  wL : Outport  Port=3
  wires:
  DCM from L to N/1(A_NL) -> To Workspace/1, A_NL/1, MatrixMultiply/2  "A_NL"
  MatrixMultiply/1 -> A_BL/1  "A_BL"
  A_BN/1 -> MatrixMultiply/1
  h_vect/1 -> Vector norm1/1(u), DCM from L to N/2(h_vect)  "h"
  Vector norm/1(u_versor) -> Terminator2/1
  r_vect/1 -> DCM from L to N/1(r_vect), Vector norm/1(u)  "r"
  Divide/1 -> Gain/1  "wL"
  Square/1 -> Divide/2
  Vector norm/2(||u||) -> Square/1
  Vector norm1/2(||u||) -> Divide/1
  Vector norm1/1(u_versor) -> Terminator1/1
  Gain/1 -> wL/1

== system Project_SADC/Sensors/Check if in EH FOV ==
  A_BN : Inport
  r_vect : Inport  Port=2
  Acos : Trigonometry  Operator=acos
  Constant : Constant  Value=[-1 0 0]
  Dot Product : DotProduct  InputSameDT=on  OutDataTypeStr=Inherit: Inherit via internal rule
  Gain : Gain  Gain=-1
  If : If  IfExpression=u1 > 90
  If Action Subsystem : Subsystem  TreatAsAtomicUnit=on
  If Action Subsystem1 : Subsystem  TreatAsAtomicUnit=on
  MatrixMultiply : Product  Multiplication=Matrix(*)
  Merge : Merge
  Radians to Degrees : simulink_extras/Transformations/Radians to Degrees
  Scope : Scope
  Terminator : Terminator
  Vector norm1 : Subsystem
  rvect _B : Outport
  wires:
  MatrixMultiply/1 -> Vector norm1/1(u)
  Vector norm1/1(u_versor) -> If Action Subsystem1/1(u_versor), If Action Subsystem/1(u_versor), Dot Product/1
  Radians to Degrees/1 -> If/1, Scope/1
  Merge/1 -> rvect _B/1
  If Action Subsystem/1(Out1) -> Merge/1
  If Action Subsystem1/1(Out1) -> Merge/2
  If/2 -> If Action Subsystem1/Action
  If/1 -> If Action Subsystem/Action
  Constant/1 -> Dot Product/2
  Acos/1 -> Radians to Degrees/1
  Dot Product/1 -> Acos/1
  Vector norm1/2(||u||) -> Terminator/1
  A_BN/1 -> MatrixMultiply/1
  Gain/1 -> MatrixMultiply/2  "r_vect_in_N"
  r_vect/1 -> Gain/1

== system Project_SADC/Sensors/Check if in sunsensor FOV ==
  rSun_N : Inport
  A_BN : Inport  Port=2
  r_vect : Inport  Port=3
  Acos : Trigonometry  Operator=acos
  Constant : Constant  Value=[1 0 0]
  Dot Product : DotProduct  InputSameDT=on  OutDataTypeStr=Inherit: Inherit via internal rule
  Gain : Gain  Gain=-1
  If : If  IfExpression=u1 > 60
  If Action Subsystem : Subsystem  TreatAsAtomicUnit=on
  If Action Subsystem1 : Subsystem  TreatAsAtomicUnit=on
  MatrixMultiply : Product  Multiplication=Matrix(*)
  MatrixMultiply1 : Product  Multiplication=Matrix(*)
  Merge : Merge
  Radians to Degrees : simulink_extras/Transformations/Radians to Degrees
  Scope : Scope
  Sum : Sum  Inputs=|++
  Terminator : Terminator
  Vector norm1 : Subsystem
  Sun_B : Outport
  rSun_B : Outport  Port=2
  wires:
  r_vect/1 -> Gain/1
  Sum/1 -> MatrixMultiply/2  "r_sun_sc_in_N"
  A_BN/1 -> MatrixMultiply1/1, MatrixMultiply/1
  Vector norm1/2(||u||) -> Terminator/1
  MatrixMultiply/1 -> Vector norm1/1(u)
  Dot Product/1 -> Acos/1
  Acos/1 -> Radians to Degrees/1
  Constant/1 -> Dot Product/2
  rSun_N/1 -> MatrixMultiply1/2, Sum/1
  Gain/1 -> Sum/2
  If/1 -> If Action Subsystem/Action
  If/2 -> If Action Subsystem1/Action
  If Action Subsystem1/1(Out1) -> Merge/2
  If Action Subsystem/1(Out1) -> Merge/1
  Merge/1 -> rSun_B/1
  Radians to Degrees/1 -> Scope/1, If/1
  Vector norm1/1(u_versor) -> Dot Product/1
  MatrixMultiply1/1 -> Sun_B/1, If Action Subsystem1/1(In1), If Action Subsystem/1(In1)

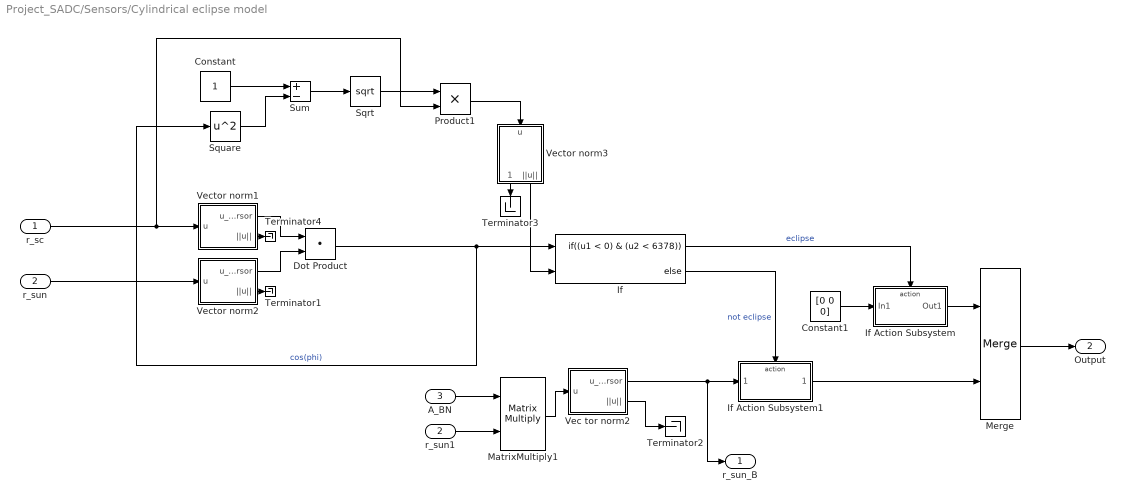
== system Project_SADC/Sensors/Cylindrical eclipse model ==
  r_sc : Inport
  r_sun : Inport  Port=2
  A_BN : Inport  Port=3
  Constant : Constant
  Constant1 : Constant  Value=[0 0 0]
  Dot Product : DotProduct  InputSameDT=on  OutDataTypeStr=Inherit: Inherit via internal rule
  If : If  NumInputs=2  IfExpression=(u1 < 0) & (u2 < 6378)
  If Action Subsystem : Subsystem  TreatAsAtomicUnit=on
  If Action Subsystem1 : Subsystem  TreatAsAtomicUnit=on
  MatrixMultiply1 : Product  Multiplication=Matrix(*)
  Merge : Merge
  Product1 : Product
  Sqrt : Sqrt  SaturateOnIntegerOverflow=on
  Square : Math  Operator=square  SaturateOnIntegerOverflow=on
  Sum : Sum  Inputs=+-
  Terminator{1..4} (4 alike) : Terminator
  Vec tor norm2 : Subsystem
  Vector norm1 : Subsystem
  Vector norm2 : Subsystem
  Vector norm3 : Subsystem
  r_sun1 : InportShadow  Port=2
  r_sun_B : Outport
  Output : Outport  Port=2
  wires:
  r_sc/1 -> Product1/2, Vector norm1/1(u)
  r_sun/1 -> Vector norm2/1(u)
  Dot Product/1 -> Square/1, If/1  "cos(phi)"
  Constant/1 -> Sum/1
  Square/1 -> Sum/2
  Sum/1 -> Sqrt/1
  Sqrt/1 -> Product1/1
  If/1 -> If Action Subsystem/Action  "eclipse"
  If/2 -> If Action Subsystem1/Action  "not eclipse"
  Constant1/1 -> If Action Subsystem/1(In1)
  If Action Subsystem1/1(Output1) -> Merge/2
  If Action Subsystem/1(Out1) -> Merge/1
  Merge/1 -> Output/1
  Product1/1 -> Vector norm3/1(u)
  Vector norm3/2(||u||) -> If/2
  Vector norm3/1(u_versor) -> Terminator3/1
  MatrixMultiply1/1 -> Vec tor norm2/1(u)
  r_sun1/1 -> MatrixMultiply1/2
  Vec tor norm2/1(u_versor) -> r_sun_B/1, If Action Subsystem1/1(u_versor)
  Vec tor norm2/2(||u||) -> Terminator2/1
  A_BN/1 -> MatrixMultiply1/1
  Vector norm1/1(u_versor) -> Dot Product/1
  Vector norm2/1(u_versor) -> Dot Product/2
  Vector norm1/2(||u||) -> Terminator4/1
  Vector norm2/2(||u||) -> Terminator1/1

== system Project_SADC/Sensors/Earth horizon ==
  rEarth_B : Inport
  A_eps : Subsystem
  MatrixMultiply : Product  Multiplication=Matrix(*)
  Zero-Order Hold2 : ZeroOrderHold  SampleTime=horizonsensor.samplingtime
  Output2 : Outport
  wires:
  A_eps/1(Out1) -> MatrixMultiply/1
  MatrixMultiply/1 -> Zero-Order Hold2/1
  rEarth_B/1 -> MatrixMultiply/2
  Zero-Order Hold2/1 -> Output2/1

== system Project_SADC/Sensors/Gyroscope ==
  wb : Inport
  Gyroscope1 : Subsystem
  Scope : Scope  NumInputPorts=2
  w_sens : Outport
  wires:
  Gyroscope1/1(w_sens) -> Scope/2, w_sens/1
  wb/1 -> Scope/1, Gyroscope1/1(w_b)

== system Project_SADC/Sensors/Magnetosensor ==
  b_B : Inport
  Constant : Constant  Value=magnetometer.A_eps
  Constant1 : Constant  Value=magnetometer.noise
  MatrixMultiply : Product  Multiplication=Matrix(*)
  Saturation : Saturate  UpperLimit=magnetometer.maxval  LowerLimit=magnetometer.minval
  Scope : Scope  NumInputPorts=2
  Sum : Sum
  Zero-Order Hold1 : ZeroOrderHold  SampleTime=magnetometer.samplingtime
  b_measured : Outport
  wires:
  Sum/1 -> MatrixMultiply/2
  Constant1/1 -> Sum/1
  Constant/1 -> MatrixMultiply/1
  MatrixMultiply/1 -> Scope/1, Saturation/1
  Saturation/1 -> Zero-Order Hold1/1, Scope/2
  b_B/1 -> Sum/2
  Zero-Order Hold1/1 -> b_measured/1

== system Project_SADC/Sensors/Sun sensor ==
  rSun_B : Inport
  A_eps : Subsystem
  MatrixMultiply : Product  Multiplication=Matrix(*)
  Zero-Order Hold2 : ZeroOrderHold  SampleTime=sunsensor.samplingtime
  Output1 : Outport
  wires:
  A_eps/1(Out1) -> MatrixMultiply/1
  MatrixMultiply/1 -> Zero-Order Hold2/1
  rSun_B/1 -> MatrixMultiply/2
  Zero-Order Hold2/1 -> Output1/1

== system Project_SADC/Attitude determination /A determination/If Action Subsystem ==
  In1 : Inport
  Action Port : ActionPort  ActionPortLabel=if(u1 == 2)
  Out1 : Outport
  wires:
  In1/1 -> Out1/1

== system Project_SADC/Attitude determination /A determination/If Action Subsystem1 ==
  A : Inport
  Action Port : ActionPort  ActionPortLabel=else
  Out1 : Outport
  wires:
  A/1 -> Out1/1

== system Project_SADC/Attitude determination /State Observer/Subsystem ==
  vect : Inport
  Add : Sum  Inputs=+++
  Demux : Demux  Outputs=3
  Gain : Gain  Gain=[0 0 0; 0 0 -1; 0 1 0]
  Gain1 : Gain  Gain=[0 0 1; 0 0 0; -1 0 0]
  Gain2 : Gain  Gain=[0 -1 0; 1 0 0; 0 0 0]
  skew_mat : Outport
  wires:
  Gain1/1 -> Add/2
  Add/1 -> skew_mat/1
  Demux/3 -> Gain2/1
  Demux/1 -> Gain/1
  Demux/2 -> Gain1/1
  vect/1 -> Demux/1
  Gain/1 -> Add/1
  Gain2/1 -> Add/3

== system Project_SADC/Attitude determination /TRIAD /Vector norm1 ==
  u : Inport
  Divide : Product  Inputs=*/
  norm_vector : Subsystem
  u_versor : Outport
  ||u|| : Outport  Port=2
  wires:
  u/1 -> Divide/1, norm_vector/1(u)
  norm_vector/1(|u|) -> ||u||/1, Divide/2
  Divide/1 -> u_versor/1

== system Project_SADC/Attitude determination /TRIAD /Vector norm2 ==
  u : Inport
  Divide : Product  Inputs=*/
  norm_vector : Subsystem
  u_versor : Outport
  ||u|| : Outport  Port=2
  wires:
  u/1 -> Divide/1, norm_vector/1(u)
  norm_vector/1(|u|) -> ||u||/1, Divide/2
  Divide/1 -> u_versor/1

== system Project_SADC/Attitude determination /TRIAD /product vector2 ==
  A : Inport
  B : Inport  Port=2
  Mux : Mux  Inputs=3
  i-component : Subsystem
  j-component : Subsystem
  k-component1 : Subsystem
  C : Outport
  wires:
  k-component1/1(Out1) -> Mux/3
  j-component/1(Out1) -> Mux/2
  i-component/1(Out2) -> Mux/1
  B/1 -> i-component/2(B), j-component/2(B), k-component1/2(B)
  A/1 -> i-component/1(A), j-component/1(A), k-component1/1(A)
  Mux/1 -> C/1

== system Project_SADC/Attitude determination /TRIAD /product vector3 ==
  A : Inport
  B : Inport  Port=2
  Mux : Mux  Inputs=3
  i-component : Subsystem
  j-component : Subsystem
  k-component1 : Subsystem
  C : Outport
  wires:
  Mux/1 -> C/1
  A/1 -> k-component1/1(A), j-component/1(A), i-component/1(A)
  B/1 -> k-component1/2(B), j-component/2(B), i-component/2(B)
  i-component/1(Out2) -> Mux/1
  j-component/1(Out1) -> Mux/2
  k-component1/1(Out1) -> Mux/3

== system Project_SADC/Attitude determination /TRIAD /product vector4 ==
  A : Inport
  B : Inport  Port=2
  Mux : Mux  Inputs=3
  i-component : Subsystem
  j-component : Subsystem
  k-component1 : Subsystem
  C : Outport
  wires:
  Mux/1 -> C/1
  A/1 -> k-component1/1(A), j-component/1(A), i-component/1(A)
  B/1 -> k-component1/2(B), j-component/2(B), i-component/2(B)
  i-component/1(Out2) -> Mux/1
  j-component/1(Out1) -> Mux/2
  k-component1/1(Out1) -> Mux/3

== system Project_SADC/Attitude determination /TRIAD /product vector5 ==
  A : Inport
  B : Inport  Port=2
  Mux : Mux  Inputs=3
  i-component : Subsystem
  j-component : Subsystem
  k-component1 : Subsystem
  C : Outport
  wires:
  k-component1/1(Out1) -> Mux/3
  j-component/1(Out1) -> Mux/2
  i-component/1(Out2) -> Mux/1
  B/1 -> i-component/2(B), j-component/2(B), k-component1/2(B)
  A/1 -> i-component/1(A), j-component/1(A), k-component1/1(A)
  Mux/1 -> C/1

== system Project_SADC/Attitude determination /Vector norm1/norm_vector ==
  u : Inport
  Demux : Demux  Outputs=3
  Square : Math  Operator=square  SaturateOnIntegerOverflow=on
  Square Root : Sqrt  SaturateOnIntegerOverflow=on
  Square1 : Math  Operator=square  SaturateOnIntegerOverflow=on
  Square3 : Math  Operator=square  SaturateOnIntegerOverflow=on
  Sum : Sum  Inputs=+++
  |u| : Outport
  wires:
  u/1 -> Demux/1
  Demux/1 -> Square/1
  Demux/2 -> Square1/1
  Demux/3 -> Square3/1
  Square/1 -> Sum/1
  Square3/1 -> Sum/3
  Square1/1 -> Sum/2
  Sum/1 -> Square Root/1
  Square Root/1 -> |u|/1

== system Project_SADC/Attitude determination /Vector norm4/norm_vector ==
  u : Inport
  Demux : Demux  Outputs=3
  Square : Math  Operator=square  SaturateOnIntegerOverflow=on
  Square Root : Sqrt  SaturateOnIntegerOverflow=on
  Square1 : Math  Operator=square  SaturateOnIntegerOverflow=on
  Square3 : Math  Operator=square  SaturateOnIntegerOverflow=on
  Sum : Sum  Inputs=+++
  |u| : Outport
  wires:
  u/1 -> Demux/1
  Demux/1 -> Square/1
  Demux/2 -> Square1/1
  Demux/3 -> Square3/1
  Square/1 -> Sum/1
  Square3/1 -> Sum/3
  Square1/1 -> Sum/2
  Sum/1 -> Square Root/1
  Square Root/1 -> |u|/1

== system Project_SADC/Attitude determination /Vector norm5/norm_vector ==
  u : Inport
  Demux : Demux  Outputs=3
  Square : Math  Operator=square  SaturateOnIntegerOverflow=on
  Square Root : Sqrt  SaturateOnIntegerOverflow=on
  Square1 : Math  Operator=square  SaturateOnIntegerOverflow=on
  Square3 : Math  Operator=square  SaturateOnIntegerOverflow=on
  Sum : Sum  Inputs=+++
  |u| : Outport
  wires:
  Square Root/1 -> |u|/1
  Sum/1 -> Square Root/1
  Square1/1 -> Sum/2
  Square3/1 -> Sum/3
  Square/1 -> Sum/1
  Demux/3 -> Square3/1
  Demux/2 -> Square1/1
  Demux/1 -> Square/1
  u/1 -> Demux/1

== system Project_SADC/Attitude determination /Vector norm6/norm_vector ==
  u : Inport
  Demux : Demux  Outputs=3
  Square : Math  Operator=square  SaturateOnIntegerOverflow=on
  Square Root : Sqrt  SaturateOnIntegerOverflow=on
  Square1 : Math  Operator=square  SaturateOnIntegerOverflow=on
  Square3 : Math  Operator=square  SaturateOnIntegerOverflow=on
  Sum : Sum  Inputs=+++
  |u| : Outport
  wires:
  u/1 -> Demux/1
  Demux/1 -> Square/1
  Demux/2 -> Square1/1
  Demux/3 -> Square3/1
  Square/1 -> Sum/1
  Square3/1 -> Sum/3
  Square1/1 -> Sum/2
  Sum/1 -> Square Root/1
  Square Root/1 -> |u|/1

== system Project_SADC/Attitude determination /selection sensor/If Action Subsystem ==
  Earth_horizon : Inport
  Action Port : ActionPort
  Out1 : Outport
  wires:
  Earth_horizon/1 -> Out1/1

== system Project_SADC/Attitude determination /selection sensor/If Action Subsystem1 ==
  Sun_sensor : Inport
  Action Port : ActionPort
  Out1 : Outport
  wires:
  Sun_sensor/1 -> Out1/1

== system Project_SADC/Attitude determination /selection sensor/If Action Subsystem2 ==
  r_vect : Inport
  Action Port : ActionPort
  Out1 : Outport
  wires:
  r_vect/1 -> Out1/1
